simulink model "main"  (R2021a)
settings: Solver=FixedStepDiscrete  StartTime=0  StopTime=20  FixedStep=0.1  RelTol=1e-3
PreLoadFcn:
  | preloadFcn
values from neighbouring files (symbols this model uses):
  egoTargetSpd_kph = 60    [preloadFcn.m]
  iniEgoHeading = egoInfo(1,3)    [preloadFcn.m]
  iniEgoPos = egoInfo(1,1:2)    [preloadFcn.m]
  iniEgoSpd = egoInfo(1,4:5)    [preloadFcn.m]
  iniObsHeading1 = refInfo_obs1(1,3)    [preloadFcn.m]
  iniObsHeading2 = refInfo_obs2(1,3)    [preloadFcn.m]
  iniObsPos1 = refInfo_obs1(1,1:2)    [preloadFcn.m]
  iniObsPos2 = refInfo_obs2(1,1:2)    [preloadFcn.m]
  iniObsSpd1 = refInfo_obs1(1,4:5)    [preloadFcn.m]
  iniObsSpd2 = refInfo_obs2(1,4:5)    [preloadFcn.m]
  mu = [-2.06408447904 -1.49508472185]    [dataSet.mat]
  sig = [50.3880002876 29.2458553231]    [dataSet.mat]
undefined symbols (not defined in the file or in its folder): leftWaypoints, refInfo_obs1, refInfo_obs2, rightWaypoints
libraries: deeplib x2, fuzblock x1
(part 1 of 2)
settings Model: Creator=Ally  LastModifiedBy=Ally

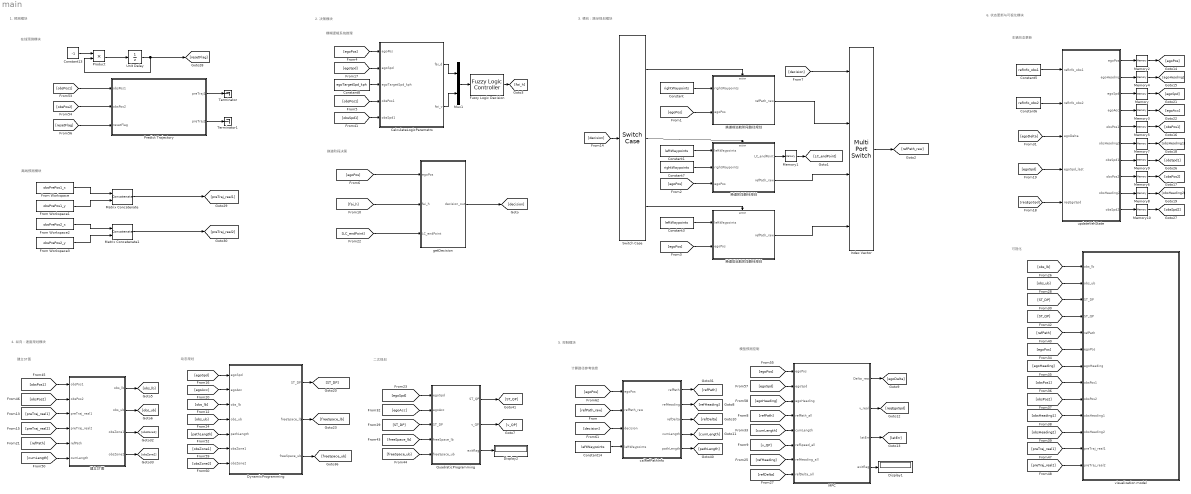
== system main ==
  note: 可视化
  note: 车辆状态更新
  note: 模型预测控制
  note: 计算路径参考信息
  note: 二次规划
  note: 动态规划
  note: 建立ST图
  note: 换道阶段决策
  note: 模糊逻辑系统推理
  note: 在线预测模块
  note: 离线预测模块
  note: 6. 状态更新与可视化模块
  note: 5. 控制模块
  note: 4. 纵向：速度规划模块
  note: 3. 横向：路径规划模块
  note: 2. 决策模块
  note: 1. 预测模块
  CalculateLogicParemetrs : MATLAB Function  TreatAsAtomicUnit=on
  Constant : Constant  Value=rightWaypoints
  Constant1 : Constant  Value=leftWaypoints
  Constant13 : Constant  Value=-1
  Constant14 : Constant  Value=leftWaypoints
  Constant3 : Constant  Value=leftWaypoints
  Constant5 : Constant  Value=refInfo_obs1
  Constant6 : Constant  Value=refInfo_obs2
  Constant7 : Constant  Value=rightWaypoints
  Constant8 : Constant  Value=egoTargetSpd_kph
  Display1 : Display
  Display2 : Display
  DynamicProgramming : MATLAB Function  TreatAsAtomicUnit=on
  From Workspace : FromWorkspace  VariableName=obsPrePos1_x
  From Workspace1 : FromWorkspace  VariableName=obsPrePos1_y
  From Workspace2 : FromWorkspace  VariableName=obsPrePos2_x
  From Workspace3 : FromWorkspace  VariableName=obsPrePos2_y
  Fuzzy Logic Decision : fuzblock/Fuzzy Logic  Controller  FIS='LCD.fis'  OutputSampleNumber=101  DataType=double  FuzzifiedInputs=off  RuleFiringStrengths=off  RuleOutputs=off  AggregatedOutputs=off  SimulateUsing=Interpreted execution  OutOfRangeInputValueMessage=warning  NoRuleFiredMessage=warning  EmptyOutputFuzzySetMessage=warning
  Index Vector : MultiPortSwitch
  MPC : MATLAB Function  TreatAsAtomicUnit=on
  Matrix Concatenate : Concatenate  Mode=Multidimensional array  ConcatenateDimension=2
  Matrix Concatenate1 : Concatenate  Mode=Multidimensional array  ConcatenateDimension=2
  Memory : Memory  InitialCondition=iniEgoSpd
  Memory1 : Memory  InitialCondition=[0 0]
  Memory10 : Memory  InitialCondition=iniObsSpd2
  Memory2 : Memory  InitialCondition=iniEgoPos
  Memory3 : Memory
  Memory4 : Memory  InitialCondition=iniEgoHeading
  Memory5 : Memory  InitialCondition=iniObsPos1
  Memory6 : Memory  InitialCondition=iniObsPos2
  Memory7 : Memory  InitialCondition=iniObsHeading1
  Memory8 : Memory  InitialCondition=iniObsHeading2
  Memory9 : Memory  InitialCondition=iniObsSpd1
  Mux1 : Mux  Inputs=2
  Predict Trajectory : Subsystem  TreatAsAtomicUnit=on
  Product : Product
  QuadraticProgramming : MATLAB Function  TreatAsAtomicUnit=on
  Switch Case : SwitchCase  CaseConditions={1,2,3}  ShowDefaultCase=off
  Terminator : Terminator
  Terminator1 : Terminator
  Unit Delay : UnitDelay  InitialCondition=1  SampleTime=-1  HasFrameUpgradeWarning=on
  calRefPathInfo : MATLAB Function  TreatAsAtomicUnit=on
  getDecision : MATLAB Function  TreatAsAtomicUnit=on
  updateVehState : MATLAB Function  TreatAsAtomicUnit=on
  visualization model : MATLAB Function  TreatAsAtomicUnit=on
  建立ST图 : MATLAB Function  TreatAsAtomicUnit=on
  换道前巡航阶段路径规划 : Subsystem  TreatAsAtomicUnit=on
  换道后巡航阶段路径规划 : Subsystem  TreatAsAtomicUnit=on
  换道阶段路径规划 : Subsystem  TreatAsAtomicUnit=on
  wires:
  CalculateLogicParemetrs/1(fai_d) -> Mux1/1
  [egoPos] -> CalculateLogicParemetrs/1(egoPos)
  getDecision/1(decision_out) -> [decision]
  CalculateLogicParemetrs/2(fai_v) -> Mux1/2
  [egoSpd] -> CalculateLogicParemetrs/2(egoSpd)
  [LC_endPoint] -> getDecision/3(LC_endPoint)
  Mux1/1 -> Fuzzy Logic Decision/1
  Switch Case/2 -> 换道阶段路径规划/Action
  Switch Case/1 -> 换道前巡航阶段路径规划/Action
  [decision] -> Switch Case/1
  Constant/1 -> 换道前巡航阶段路径规划/1(rightWaypoints)
  [egoPos] -> 换道前巡航阶段路径规划/2(egoPos)
  Constant1/1 -> 换道阶段路径规划/1(leftWaypoints)
  [egoPos] -> 换道后巡航阶段路径规划/2(egoPos)
  Constant3/1 -> 换道后巡航阶段路径规划/1(leftWaypoints)
  Switch Case/3 -> 换道后巡航阶段路径规划/Action
  换道前巡航阶段路径规划/1(refPath_raw) -> Index Vector/2
  换道后巡航阶段路径规划/1(refPath_raw) -> Index Vector/4
  [decision] -> Index Vector/1
  Index Vector/1 -> [refPath_raw]
  [preTraj_real1] -> 建立ST图/3(preTraj_real1)
  [preTraj_real2] -> 建立ST图/4(preTraj_real2)
  [refPath] -> 建立ST图/5(refPath)
  建立ST图/1(obs_lb) -> [obs_lb]
  建立ST图/2(obs_ub) -> [obs_ub]
  [obs_lb] -> DynamicProgramming/3(obs_lb)
  [obs_ub] -> DynamicProgramming/4(obs_ub)
  QuadraticProgramming/2(v_QP) -> [v_QP]
  [refPath_raw] -> calRefPathInfo/2(refPath_raw)
  calRefPathInfo/2(refHeading) -> [refHeading]
  calRefPathInfo/3(refDelta) -> [refDelta]
  calRefPathInfo/4(cumLength) -> [cumLength]
  [refPath] -> MPC/4(refPath_all)
  [v_QP] -> MPC/6(refSpeed_all)
  [refHeading] -> MPC/7(refHeading_all)
  [refDelta] -> MPC/8(refDelta_all)
  MPC/1(Delta_real) -> [egoDelta]
  MPC/3(latErr) -> [latErr]
  Constant5/1 -> updateVehState/1(refInfo_obs1)
  Constant6/1 -> updateVehState/2(refInfo_obs2)
  [egoDelta] -> updateVehState/3(egoDelta)
  [reqEgoSpd] -> updateVehState/5(reqEgoSpd)
  updateVehState/1(egoPos) -> Memory2/1
  updateVehState/2(egoHeading) -> Memory4/1
  updateVehState/5(obsPos1) -> Memory5/1
  updateVehState/8(obsPos2) -> Memory6/1
  updateVehState/6(obsHeading1) -> Memory7/1
  updateVehState/9(obsHeading2) -> Memory8/1
  [obs_lb] -> visualization model/1(obs_lb)
  [obs_ub] -> visualization model/2(obs_ub)
  DynamicProgramming/1(ST_DP) -> [ST_DP]
  [ST_DP] -> QuadraticProgramming/3(ST_DP)
  [ST_DP] -> visualization model/3(ST_DP)
  [ST_QP] -> visualization model/4(ST_QP)
  [refPath] -> visualization model/5(refPath)
  [egoPos] -> visualization model/6(egoPos)
  [egoHeading] -> visualization model/7(egoHeading)
  [obsPos1] -> visualization model/8(obsPos1)
  [obsPos2] -> visualization model/9(obsPos2)
  [obsHeading1] -> visualization model/10(obsHeading1)
  [obsHeading2] -> visualization model/11(obsHeading2)
  [egoPos] -> 换道阶段路径规划/3(egoPos)
  [egoPos] -> getDecision/1(egoPos)
  MPC/2(v_real) -> [reqEgoSpd]
  updateVehState/3(egoSpd) -> Memory/1
  updateVehState/4(egoAcc) -> Memory3/1
  Memory/1 -> [egoSpd]
  [egoSpd] -> updateVehState/4(egoSpd_last)
  updateVehState/7(obsSpd1) -> Memory9/1
  updateVehState/10(obsSpd2) -> Memory10/1
  Constant8/1 -> CalculateLogicParemetrs/3(egoTargetSpd_kph)
  [obsPos1] -> CalculateLogicParemetrs/4(obsPos1)
  [obsSpd1] -> CalculateLogicParemetrs/5(obsSpd1)
  Memory1/1 -> [LC_endPoint]
  Memory2/1 -> [egoPos]
  Memory3/1 -> [egoAcc]
  Memory4/1 -> [egoHeading]
  Memory5/1 -> [obsPos1]
  Memory6/1 -> [obsPos2]
  Memory7/1 -> [obsHeading1]
  Memory8/1 -> [obsHeading2]
  Memory9/1 -> [obsSpd1]
  Memory10/1 -> [obsSpd2]
  Constant7/1 -> 换道阶段路径规划/2(rightWaypoints)
  [egoSpd] -> DynamicProgramming/1(egoSpd)
  [egoAcc] -> DynamicProgramming/2(egoAcc)
  [egoAcc] -> QuadraticProgramming/2(egoAcc)
  DynamicProgramming/2(freeSpace_lb) -> [freeSpace_lb]
  DynamicProgramming/3(freeSpace_ub) -> [freeSpace_ub]
  [freeSpace_lb] -> QuadraticProgramming/4(freeSpace_lb)
  [freeSpace_ub] -> QuadraticProgramming/5(freeSpace_ub)
  [egoSpd] -> QuadraticProgramming/1(egoSpd)
  QuadraticProgramming/3(exitflag) -> Display2/1
  calRefPathInfo/5(pathLength) -> [pathLength]
  [cumLength] -> 建立ST图/6(cumLength)
  [pathLength] -> DynamicProgramming/5(pathLength)
  MPC/4(exitflag) -> Display1/1
  QuadraticProgramming/1(ST_QP) -> [ST_QP]
  [cumLength] -> MPC/5(cumLength)
  [obsPos1] -> 建立ST图/1(obsPos1)
  [obsPos2] -> 建立ST图/2(obsPos2)
  [preTraj_real1] -> visualization model/12(preTraj_real1)
  [preTraj_real2] -> visualization model/13(preTraj_real2)
  Product/1 -> Unit Delay/1
  Unit Delay/1 -> [resetFlag], Product/2
  Constant13/1 -> Product/1
  [resetFlag] -> Predict Trajectory/3(resetFlag)
  [obsPos1] -> Predict Trajectory/1(obsPos1)
  [obsPos2] -> Predict Trajectory/2(obsPos2)
  Predict Trajectory/1(preTraj1) -> Terminator/1
  Predict Trajectory/2(preTraj2) -> Terminator1/1
  From Workspace/1 -> Matrix Concatenate/1
  From Workspace1/1 -> Matrix Concatenate/2
  From Workspace2/1 -> Matrix Concatenate1/1
  From Workspace3/1 -> Matrix Concatenate1/2
  Matrix Concatenate/1 -> [preTraj_real1]
  Matrix Concatenate1/1 -> [preTraj_real2]
  [egoPos] -> MPC/1(egoPos)
  [egoSpd] -> MPC/2(egoSpd)
  [egoHeading] -> MPC/3(egoHeading)
  calRefPathInfo/1(refPath) -> [refPath]
  建立ST图/3(obsZone1) -> [obsZone1]
  建立ST图/4(obsZone2) -> [obsZone2]
  [obsZone1] -> DynamicProgramming/6(obsZone1)
  [obsZone2] -> DynamicProgramming/7(obsZone2)
  [decision] -> calRefPathInfo/3(decision)
  [egoPos] -> calRefPathInfo/1(egoPos)
  Constant14/1 -> calRefPathInfo/4(leftWaypoints)
  Fuzzy Logic Decision/1 -> [fai_h]
  [fai_h] -> getDecision/2(fai_h)
  换道阶段路径规划/1(LC_endPoint) -> Memory1/1
  换道阶段路径规划/2(refPath_raw) -> Index Vector/3

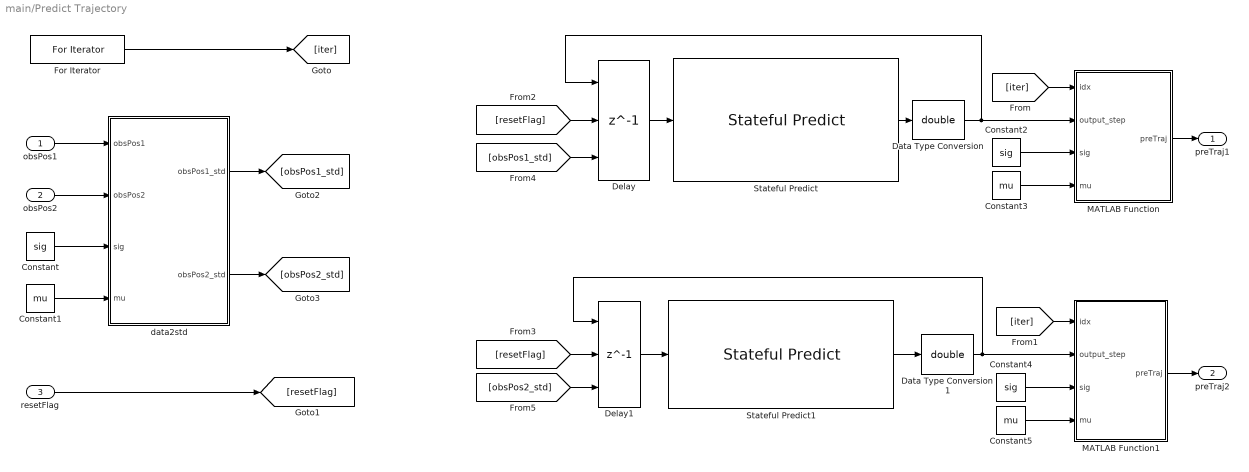
== system main/Predict Trajectory ==
  obsPos1 : Inport
  obsPos2 : Inport  Port=2
  resetFlag : Inport  Port=3
  Constant : Constant  Value=sig
  Constant1 : Constant  Value=mu
  Constant2 : Constant  Value=sig
  Constant3 : Constant  Value=mu
  Constant4 : Constant  Value=sig
  Constant5 : Constant  Value=mu
  Data Type Conversion : DataTypeConversion  OutDataTypeStr=double
  Data Type Conversion1 : DataTypeConversion  OutDataTypeStr=double
  Delay : Delay  DelayLength=1  InitialConditionSource=Input port  ExternalReset=Either
      settings: InputPortMap=u0,r5,p4
  Delay1 : Delay  DelayLength=1  InitialConditionSource=Input port  ExternalReset=Either
      settings: InputPortMap=u0,r5,p4
  For Iterator : ForIterator  IterationLimit=10
  MATLAB Function : MATLAB Function  TreatAsAtomicUnit=on
  MATLAB Function1 : MATLAB Function  TreatAsAtomicUnit=on
  Stateful Predict : deeplib/Stateful Predict  Network=Network from MAT-file  NetworkFunction=untitled  NetworkFilePath=C:\Users\Ally\Desktop\LSTM.mat  InputDataFormats={ '', '' }  SampleTime=-1  ForceInterpretedSim=off  EnableDLNetwork=on
      settings: SourceProductBaseCode=NN
  Stateful Predict1 : deeplib/Stateful Predict  Network=Network from MAT-file  NetworkFunction=untitled  NetworkFilePath=C:\Users\Ally\Desktop\LSTM.mat  InputDataFormats={ '', '' }  SampleTime=-1  ForceInterpretedSim=off  EnableDLNetwork=on
      settings: SourceProductBaseCode=NN
  data2std : MATLAB Function  TreatAsAtomicUnit=on
  preTraj1 : Outport
  preTraj2 : Outport  Port=2
  wires:
  data2std/2(obsPos2_std) -> [obsPos2_std]
  [obsPos2_std] -> Delay1/3
  data2std/1(obsPos1_std) -> [obsPos1_std]
  Constant1/1 -> data2std/4(mu)
  Stateful Predict1/1 -> Data Type Conversion1/1
  obsPos2/1 -> data2std/2(obsPos2)
  For Iterator/1 -> [iter]
  [resetFlag] -> Delay1/2
  Data Type Conversion/1 -> MATLAB Function/2(output_step), Delay/1
  Delay1/1 -> Stateful Predict1/1
  MATLAB Function/1(preTraj) -> preTraj1/1
  Data Type Conversion1/1 -> MATLAB Function1/2(output_step), Delay1/1
  Constant4/1 -> MATLAB Function1/3(sig)
  obsPos1/1 -> data2std/1(obsPos1)
  [iter] -> MATLAB Function/1(idx)
  MATLAB Function1/1(preTraj) -> preTraj2/1
  [iter] -> MATLAB Function1/1(idx)
  resetFlag/1 -> [resetFlag]
  [resetFlag] -> Delay/2
  Constant2/1 -> MATLAB Function/3(sig)
  Constant3/1 -> MATLAB Function/4(mu)
  Constant/1 -> data2std/3(sig)
  Constant5/1 -> MATLAB Function1/4(mu)
  Stateful Predict/1 -> Data Type Conversion/1
  [obsPos1_std] -> Delay/3
  Delay/1 -> Stateful Predict/1

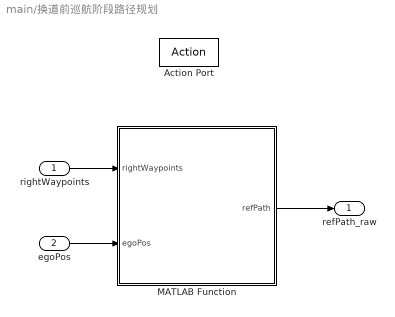
== system main/换道前巡航阶段路径规划 ==
  rightWaypoints : Inport
  egoPos : Inport  Port=2
  Action Port : ActionPort  ActionPortLabel=case [ 1 ]:
  MATLAB Function : MATLAB Function  TreatAsAtomicUnit=on
  refPath_raw : Outport  VectorParamsAs1DForOutWhenUnconnected=off
  wires:
  rightWaypoints/1 -> MATLAB Function/1(rightWaypoints)
  MATLAB Function/1(refPath) -> refPath_raw/1
  egoPos/1 -> MATLAB Function/2(egoPos)

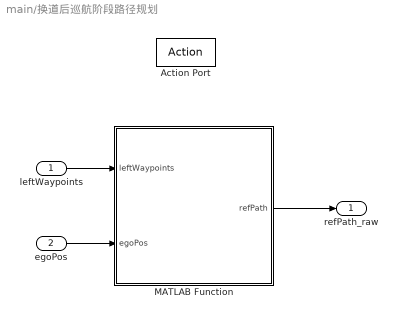
== system main/换道后巡航阶段路径规划 ==
  leftWaypoints : Inport
  egoPos : Inport  Port=2
  Action Port : ActionPort  ActionPortLabel=case [ 3 ]:
  MATLAB Function : MATLAB Function  TreatAsAtomicUnit=on
  refPath_raw : Outport  VectorParamsAs1DForOutWhenUnconnected=off
  wires:
  egoPos/1 -> MATLAB Function/2(egoPos)
  MATLAB Function/1(refPath) -> refPath_raw/1
  leftWaypoints/1 -> MATLAB Function/1(leftWaypoints)

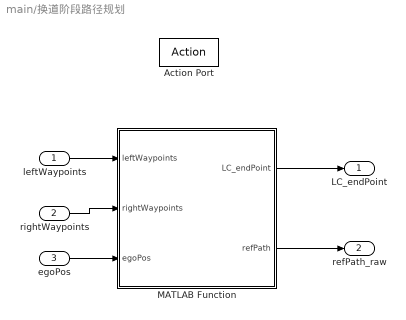
== system main/换道阶段路径规划 ==
  leftWaypoints : Inport
  rightWaypoints : Inport  Port=2
  egoPos : Inport  Port=3
  Action Port : ActionPort  ActionPortLabel=case [ 2 ]:
  MATLAB Function : MATLAB Function  TreatAsAtomicUnit=on
  LC_endPoint : Outport  VectorParamsAs1DForOutWhenUnconnected=off
  refPath_raw : Outport  Port=2  VectorParamsAs1DForOutWhenUnconnected=off
  wires:
  rightWaypoints/1 -> MATLAB Function/2(rightWaypoints)
  leftWaypoints/1 -> MATLAB Function/1(leftWaypoints)
  egoPos/1 -> MATLAB Function/3(egoPos)
  MATLAB Function/1(LC_endPoint) -> LC_endPoint/1
  MATLAB Function/2(refPath) -> refPath_raw/1

== matlab function main/CalculateLogicParemetrs ==
  data: egoPos input; fai_d output; egoSpd input; egoTargetSpd_kph input; obsPos1 input; obsSpd1 input; fai_v output
function [fai_d,fai_v] = CalculateLogicParemetrs(egoPos,egoSpd,egoTargetSpd_kph, obsPos1, obsSpd1)
deltDist = sqrt((egoPos(1)-obsPos1(1))^2 + (egoPos(2)-obsPos1(2))^2);
egoSpd_abs = sqrt(egoSpd(1)^2 + egoSpd(2)^2);
obsSpd_abs = sqrt(obsSpd1(1)^2 + obsSpd1(2)^2);

% 计算安全距离模型
D_slf = (egoSpd_abs-obsSpd_abs)^2 / 2/(0.0524*egoSpd_abs-0.1215) + 0.8509*obsSpd_abs+1.6109;

% 计算车距期望系数
D_f = D_slf + 10;    % 车距期望值
if deltDist >= D_f
    fai_d = 1;
else
    fai_d = deltDist / D_f;
end

% 计算速度差值系数
egoTargetSpd_mps = egoTargetSpd_kph / 3.6;   
if egoSpd_abs >= egoTargetSpd_mps
    fai_v = 1;
else
    fai_v = (egoSpd_abs - obsSpd_abs) / egoTargetSpd_mps;
end

== matlab function main/getDecision ==
  data: egoPos input; fai_h input; decision_out output; LC_endPoint input
function decision_out = getDecision(egoPos,fai_h,LC_endPoint)
persistent flag decision
if isempty(flag) || isempty(decision) 
    flag = 0;
    decision = 1;
end

if fai_h <= 0.5 && decision <= 1
    decision = 1;
else 
    % 计算本车位置与换道终点的距离
    dist = sqrt((egoPos(1) - LC_endPoint(1))^2 + (egoPos(2) - LC_endPoint(2))^2);
    if dist < 1 && flag == 0 || flag == 1
        decision = 3;
        flag = 1;
    else
        decision = 2;
    end
end
decision_out = decision;

== matlab function main/DynamicProgramming ==
  data: egoSpd input; egoAcc input; obs_lb input; ST_DP output; obs_ub input; freeSpace_lb output; freeSpace_ub output; pathLength input; obsZone1 input; obsZone2 input
function [ST_DP,freeSpace_lb,freeSpace_ub] = DynamicProgramming(egoSpd,egoAcc,obs_lb,obs_ub, pathLength, obsZone1, obsZone2)
%% 初始化
% 初始速度和加速度
v_ini = sqrt(egoSpd(1)^2 + egoSpd(2)^2);
a_ini = egoAcc;

% 路径长度限制在100米内
pathLength_max = 100;
pathLength = min([pathLength,pathLength_max]);

% 约束条件
v_max = 16;                % 最大速度
a_max = 3;                 % 最大加速度
omega = [0.4, 0.6];        % 加速度和加加速度权重

% 初始条件判断：若初始速度和加速度不满足上限值，则适当进行强制处理，避免后期QP规划失败
if v_ini + a_ini*1 > v_max
    v_ini = v_max;
    a_ini = 0;
end

% 定义状态空间，用于DP搜索
T = 8;                     % ST图总时间
dt = 1;                    % 时间离散步长
dS = 0.2;                  % 距离离散步长
N = round(T / dt);         % 一共N个阶段

% 构造表征s、t的状态空间
t_seq = 0:dt:T;                     % 时间离散向量
s_seq_max = 0:dS:pathLength_max;    % 最大的距离离散向量
s_seq = 0:dS:pathLength;            % 距离离散向量
rows = length(s_seq_max);           % 状态空间行数
cols = length(t_seq);               % 状态空间列数
validRows = length(s_seq);          % 有效的状态空间行数
stateSpace_t = zeros(rows,cols);
stateSpace_s = zeros(rows,cols);
for i = 1:length(s_seq_max)
    for j = 1:length(t_seq)
        row = length(s_seq_max)-i+1;
        col = j;
        stateSpace_t(row,col) = t_seq(j);
        stateSpace_s(row,col) = s_seq_max(i);
    end
end

%% 第1阶段（时刻0）的初步计算
% 遍历第2阶段，初步生成从第一阶段的起点到第二阶段的所有可能状态
state = zeros(12000,6);
stateNum = 0;
for i = rows:-1:(rows-validRows+1)
    % 计算位置、速度、加速度、加加速度
    s = stateSpace_s(i,2);
    v = s / dt;
    a = (v - v_ini) / dt;
    jerk = (a - a_ini) / dt;
    
    % 若满足速度、加速度约束，则将此状态追加到state中
    if v <= v_max && abs(a) <= a_max
        % 计算加速度和加加速度代价
        accCost = abs(a);
        jerkCost = abs(jerk);
        cost =  accCost*omega(1) + 2*jerkCost*omega(2);
        
        % 将第1阶段行索引、第2阶段行索引、位置、速度、加速度、加加速度、代价值存放在state中
        stateNum = stateNum + 1;
        state(stateNum,1:6) = [rows,i,s,v,a,cost];
    end
end

% 初始化最优序列
optSeq = cell(1000,1);     % 每一阶段至第1阶段的累计最优序列
for i = 1:1000
    optSeq{i,1} = zeros(9,6);
end
for i = 1:stateNum
    optSeq{i,1}(1,:) = state(i,:);
end

%% 从第2阶段（时刻dt）逐步遍历寻优
lastState = state;          % 将上面第1阶段获得的备选可行状态赋值给lastState

% 第1层循环：第i个阶段
for i = 2:N+1
    % 时间和下一可行状态初始化
    t = i-1;
    nextStateTemp = zeros(12000,6);
    stateNum_i = 1;
    lastStateNum = sum(lastState(:,1)~=0);
    
    % 第2层循环：当前第i阶段的第j个可能状态
    for j = 1:lastStateNum
        state_j = zeros(1000,6);
        stateNum_j = 0;
        lastStepIdx = lastState(j,2);
        
        %  第3层循环：第i+1阶段的第k个可能状态
        for k = lastStepIdx:-1:(rows-validRows+1)
            % 计算位置、速度、加速度、加加速度
            s = stateSpace_s(k,(i-1));
            v = (s - lastState(j,3)) / dt;
            a = (v -  lastState(j,4)) / dt;
            jerk = (a -  lastState(j,5)) / dt;
            
            % 若满足速度、加速度、障碍物约束，则将此状态追加到state_j中
            pt1 = [t+1,s];
            pt2 = [t, lastState(j,3)];
            flag = isIN(pt1, pt2, obsZone1,obsZone2);

            if flag == 0 &&  v <= v_max && abs(a) <= a_max
                % 计算代价函数
                accCost = abs(a);
                jerkCost = abs(jerk);
                cost =  accCost*omega(1) + 2*jerkCost*omega(2);
                
                % 将第i阶段行索引、第i+1阶段行索引、位置、速度、加速度、加加速度、代价值存放在state中
                stateNum_j = stateNum_j + 1;
                state_j(stateNum_j,1:6) = [lastStepIdx,k,s,v,a,cost];
            end
        end
        nextStateTemp(stateNum_i:stateNum_i+stateNum_j-1,:) = state_j(1:stateNum_j,:);
        stateNum_i = stateNum_i + stateNum_j;
    end
    
    % 故障判断：若nextStateTemp为空，表明下阶段已无任何可行状态，则执行下一个循环
    if sum(nextStateTemp(:,1)) ~= 0
        % 先将下一阶段的可行状态排序，然后只取非重复行索引序号放进s_Temp
        [~,sortIdx] = sort(nextStateTemp(:,2));
        nextStateTemp = nextStateTemp(sortIdx,:);
        s_Temp = zeros(500,1);
        uniqueNum = length(unique(nextStateTemp(:,2)));
        s_Temp(1:uniqueNum) = unique(nextStateTemp(:,2));
        
        % 由于从第i阶段的若干状态到第i+1阶段的某个状态可能有多个选择，那么应该择优处理
        nextState = zeros(12000,6);
        stateNum = 0;
        for j = 1:uniqueNum
            s = s_Temp(j);                                % 第i+1阶段的s值
            idx = find(nextStateTemp(:,2) == s);          % 找出到底有多少个重复的s值
            [~,minIdx] = min(nextStateTemp(idx,6));       % 若有多个，选择从i阶段到i+1阶段的s值的代价最小的那一个
            stateNum = stateNum + 1;
            nextState(stateNum,:) = nextStateTemp(idx(minIdx),:);
        end
        
        % 将本阶段的所有最优状态序列添加至opt_seq中
        opt_seq_temp = cell(1000,1);     % 每一阶段至第1阶段的累计最优序列
        for j = 1:1000
            opt_seq_temp{j,1} = zeros(9,6);
        end
        for j = 1:stateNum
            lastStepIdx = nextState(j,1);   %来自于上一个阶段的哪一个状态
            for k = 1:size(optSeq,1)
                row_optSeq_k = sum(optSeq{k,1}(:,1)~=0);
                if row_optSeq_k ~= 0 && optSeq{k,1}(row_optSeq_k,2) == lastStepIdx
                    opt_seq_temp{j,1}(1:row_optSeq_k+1,:) = [optSeq{k,1}(1:row_optSeq_k,:);
                        nextState(j,:)];
                    break
                end
            end
        end
        for j = 1:1000
            if j <= stateNum
                optSeq{j,1} = opt_seq_temp{j,1};
            else
                optSeq{j,1} =  zeros(9,6);
            end
        end
        lastState = nextState;
    end
end

%% 找出最优ST曲线
t_opt = (0:1:8)';
s_opt = [0;optSeq{2,1}(1:8,3)];
for i = 2:N+1
    if s_opt(i) == 0
        s_opt(i) = s_opt(i-1);
    end
end
ST_DP = [t_opt, s_opt];

%% 根据DP得到的ST_opt，更新上下界
freeSpace_lb = zeros(N*10,1);
freeSpace_ub = zeros(N*10,1);
for i = 1:size(ST_DP,1)-1
    s_now = ST_DP(i);
    s_next = ST_DP(i+1);
    for j = 1:10
        s = (s_next - s_now)*j/10 + s_now;
        bound = [obs_lb((i-1)*10+j,2:3), obs_ub((i-1)*10+j,2:3), s];
        temp = sort(bound);
        idx = find(temp == s);
        if idx == 1
            freeSpace_lb((i-1)*10+j) = -1000;
            freeSpace_ub((i-1)*10+j) = temp(2);
        elseif  idx == 5
            freeSpace_lb((i-1)*10+j) = temp(4);
            freeSpace_ub((i-1)*10+j) = 1000;
        else
            freeSpace_lb((i-1)*10+j) = temp(idx-1);
            freeSpace_ub((i-1)*10+j) = temp(idx+1);
        end
    end
end
idx1 = freeSpace_lb == inf;
idx2 = freeSpace_lb == -inf;
freeSpace_lb(idx1) = 1000;
freeSpace_lb(idx2) = -1000;
idx1 = freeSpace_ub == inf;
idx2 = freeSpace_ub == -inf;
freeSpace_ub(idx1) = 1000;
freeSpace_ub(idx2) = -1000;


end

%% 函数
function flag = isIN(pt1, pt2, obsZone1,obsZone2)
x = linspace(pt1(1),pt2(1),10);
y = linspace(pt1(2),pt2(2),10);

num1 = sum(obsZone1(:,1) ~= 0);
num2 = sum(obsZone2(:,1) ~= 0);
if num1 >= 4
    temp1 = double(inpolygon(x, y, obsZone1(1:num1,1), obsZone1(1:num1,2)));
else
    temp1 = zeros(1,10);
end
if num2 >= 4
    temp2 = double(inpolygon(x, y, obsZone2(1:num2,1), obsZone2(1:num2,2)));
else
    temp2 = zeros(1,10);
end
if sum(temp1) == 0 && sum(temp2) == 0
    flag = 0;
else
    flag = 1;
end
end

== matlab function main/MPC ==
  data: egoPos input; egoSpd input; egoHeading input; refPath_all input; cumLength input; refSpeed_all input size=[81,2]; Delta_real output; v_real output; refHeading_all input; refDelta_all input; latErr output; exitflag output
function [Delta_real,v_real,latErr,exitflag] = MPC(egoPos, egoSpd, egoHeading, refPath_all,cumLength, refSpeed_all, refHeading_all,refDelta_all)
%% 预处理
% 将需要跟踪的参考路径缩减为realPathNum个点即可（因为滚动跟踪，无需全部加入）
realPathNum = 10;
refPath = refPath_all(1:realPathNum,:);
refHeading = refHeading_all(1:realPathNum);
refDelta = refDelta_all(1:realPathNum);

% 对QP输出的参考速度序列进行插值获得realPathNum个点
temp = refSpeed_all(:,2) * 0.1;
cumlength_QP = cumsum(temp);
refSpeed =  zeros(1,realPathNum);
refSpeed(1) = refSpeed_all(1,2);
for i = 2:realPathNum
    s = cumLength(i);
    for j = 1:80
        if cumlength_QP(j) < s &&  cumlength_QP(j+1) > s
            refSpeed(i) = refSpeed_all(j,2);
        end
    end
end

%% 主程序
dt = 0.1;   % 时间步长
L = 2.9;    % 轴距

% 车辆初始状态定义
refPos = refPath;
iniPos = egoPos;
iniSpd = egoSpd;
iniHeading = egoHeading*pi/180;

% 赋初值
currentPos = iniPos;
currentHeading = iniHeading;

% 控制量
persistent U
if isempty(U)
    U = [0.01;0.01];
end

% 寻找预瞄距离范围内最近路径点
dist = sqrt((refPos(:,1)-currentPos(1)).^2 + (refPos(:,2)-currentPos(2)).^2);
[~,targetIdx] = min(dist);

% 调用MPC控制器
[Delta_real,v_real,latErr,U,exitflag] = MPC_controller(targetIdx,currentPos,currentHeading,refPos,refHeading,refDelta,dt,L,U,refSpeed);

end

function [Delta_real,v_real,latError,U,exitflag] = MPC_controller...
    (targetIdx,currentPos,currentHeading,refPos,refHeading,refDelta,dt,L,U,refSpeed) 

%% MPC预设参数
Nx = 3;         % 状态量的个数
Nu = 2;         % 控制量的个数
Np = 10;        % 预测步长
Nc = 10;        % 控制步长
rau = 10;       % 松弛因子
Q = 100*eye(Np*Nx);      % (Np*Nx) × (Np*Nx)
R = 1*eye(Nc*Nu);        % (Nc*Nu) × (Nc*Nu)

% 控制量约束条件
umin = [-0.2; -0.54];
umax = [0.2; 0.332];
delta_umin = [-0.05; -0.64];
delta_umax = [0.05; 0.64];

%% 原运动学误差状态空间方程的相关矩阵
% 计算参考控制量
v_r = refSpeed(targetIdx);
Delta_r = refDelta(targetIdx);
heading_r = refHeading(targetIdx);

% 实际状态量与参考状态量
X_real = [currentPos(1),currentPos(2),currentHeading];
Xr = [refPos(targetIdx,1), refPos(targetIdx,2), refHeading(targetIdx)];

% 求位置、航向角的误差
x_error  = currentPos(1) - refPos(targetIdx,1);
y_error = currentPos(2) - refPos(targetIdx,2);

% 根据百度Apolo，计算横向误差
latError = y_error*cos(heading_r) - x_error*sin(heading_r);

% a,b两个矩阵
a = [1    0   -v_r*sin(heading_r)*dt;
    0    1   v_r*cos(heading_r)*dt;
    0    0   1];
b = [cos(heading_r)*dt     0;
    sin(heading_r)*dt     0;
    tan(heading_r)*dt/L   v_r*dt/(L * (cos(Delta_r)^2))];

%% 新的状态空间方程的相关矩阵
coder.extrinsic('cell2mat');
% 新的状态量
kesi = zeros(Nx+Nu,1);              % (Nx+Nu) × 1
kesi(1:Nx) = X_real - Xr;
kesi(Nx+1:end) = U;

% 新的A矩阵
A_cell = cell(2,2);
A_cell{1,1} = a;
A_cell{1,2} = b;
A_cell{2,1} = zeros(Nu,Nx);
A_cell{2,2} = eye(Nu);
A = cell2mat(A_cell);           % (Nx+Nu) × (Nx+Nu)

% 新的B矩阵
B_cell = cell(2,1);
B_cell{1,1} = b;
B_cell{2,1} = eye(Nu);
B = cell2mat(B_cell);           % (Nx+Nu) × Nu

% 新的C矩阵
C = [eye(Nx), zeros(Nx, Nu)];   % Nx × (Nx+Nu)

% PHI矩阵
PHI_cell = cell(Np,1);
for i = 1:Np
    PHI_cell{i,1} = zeros(Nx,Nx+Nu);
    PHI_cell{i,1}=C*A^i;  % Nx × (Nx+Nu)
end
PHI = cell2mat(PHI_cell);   % (Nx * Np) × (Nx + Nu)


% THETA矩阵
THETA_cell = cell(Np,Nc);
for i = 1:Np
    for j = 1:Nc
        THETA_cell{i,j} = zeros(Nx,Nu);
        if j <= i
            THETA_cell{i,j} = C*A^(i-j)*B;    % Nx × Nu
        end
    end
end
THETA = zeros(Nx * Np,Nu * Nc);
THETA = cell2mat(THETA_cell);                 % (Nx * Np) × (Nu * Nc)

%% 二次型目标函数的相关矩阵

% 初始化H矩阵
H_cell = cell(2,2);
H_cell{1,1} = zeros(Nu*Nc, Nu*Nc);
H_cell{1,1} = THETA'*Q*THETA + R;  % (Nu * Nc) × (Nu * Nc)
H_cell{1,2} = zeros(Nu*Nc,1);
H_cell{2,1} = zeros(1,Nu*Nc);
H_cell{2,2} = rau;
H = cell2mat(H_cell);            % (Nu * Nc + 1) × (Nu * Nc + 1)

% E矩阵
E = PHI*kesi;                    % (Nx * Np) × 1

% g矩阵
g_cell = cell(2,1);
g_cell{1,1} = zeros(Nu * Nc,1);
g_cell{1,1} = E'*Q*THETA;          % (Nu * Nc ) × 1，行数为了和H的列数匹配，新添加一列0
g_cell{2,1} = 0;
g = cell2mat(g_cell);              % (Nu * Nc + 1 ) × 1

%% 约束条件的相关矩阵

% A_I矩阵
A_t = zeros(Nc,Nc);     % 下三角方阵
for i = 1:Nc
    A_t(i,1:i) = 1;
end
A_I = kron(A_t,eye(Nu));       % (Nu * Nc) × (Nu * Nc)

% Ut矩阵
Ut = kron(ones(Nc,1),U);       % (Nu * Nc) × 1

% 控制量与控制量变化量的约束
Umin = kron(ones(Nc,1),umin);
Umax = kron(ones(Nc,1),umax);
delta_Umin = kron(ones(Nc,1),delta_umin);
delta_Umax = kron(ones(Nc,1),delta_umax);

% 用于quadprog函数不等式约束Ax <= b的矩阵A
A_cons_cell = {A_I, zeros(Nu*Nc,1);       % 列数为了和H的列数匹配，新添加一列0，(Nu * Nc) × (Nu * Nc), (Nu * Nc) ×1
    -A_I, zeros(Nu*Nc,1)};
A_cons = cell2mat(A_cons_cell);           % (Nu * Nc * 2) × (Nu * Nc +1)

% 用于quadprog函数不等式约束Ax <= b的向量b
b_cons_cell = {Umax-Ut;
    -Umin+Ut};
b_cons = cell2mat(b_cons_cell);

% △U的上下界约束
lb = [delta_Umin;0];
ub = [delta_Umax;0];

%% 开始求解过程
options = optimoptions('quadprog','algorithm','active-set');
exitflag = 0;
delta_U = zeros((Nu * Nc +1),1);
x0 = zeros(Nu * Nc +1,1);
[delta_U,~,exitflag,~]  = quadprog(H,g,A_cons,b_cons,[],[],lb,ub,x0,options);   %(Nu * Nc +1) × 1

%% 计算输出

% 只选取求解的delta_U的第一组控制量。注意：这里是v_tilde的变化量和Delta_tilde的变化量
delta_v_tilde = delta_U(1);
delta_Delta_tilde = delta_U(2);

% 更新这一时刻的控制量。注意，这里的“控制量”是v_tilde和Delta_tilde，而不是真正的v和Delta
U(1) = kesi(4) + delta_v_tilde;
U(2) = kesi(5) + delta_Delta_tilde;

% 求解真正的控制量v_real和Delta_real
v_real = U(1) + v_r;
Delta_real = U(2) + Delta_r;
kk=1;
end

== matlab function main/calRefPathInfo ==
  data: egoPos input; refPath output; refPath_raw input; refHeading output; refDelta output; cumLength output; pathLength output size=1; decision input; leftWaypoints input
function [refPath,refHeading,refDelta,cumLength,pathLength] = calRefPathInfo(egoPos, refPath_raw, decision, leftWaypoints)
%% 相关参数定义
L = 2.9;    % 轴距

% 定义参考轨迹：若决策为2，表明处于换道阶段，需要对轨迹进行简单处理
if decision == 2
    % 第一部分
    deltX = refPath_raw(:,1) - egoPos(1);
    deltY = refPath_raw(:,2) - egoPos(2);
    dist = sqrt(deltX.^2 + deltY.^2);
    [~, idx1] = min(dist);
    refPath = zeros(40,2);
    refPath(1:40-idx1+1,:) = refPath_raw(idx1:40,:);
    
    % 第二部分
    if idx1 >= 2
        LC_endPoint = refPath_raw(40,:);
        deltX = leftWaypoints(:,1) - LC_endPoint(1);
        deltY = leftWaypoints(:,2) - LC_endPoint(2);
        dist = sqrt(deltX.^2 + deltY.^2);
        [~, idx2] = min(dist);
        refPath(40-idx1+2:40,:) = leftWaypoints(idx2+1 :idx1+idx2-1,1:2);
    end
else
    refPath = refPath_raw;
end
    
% 计算航向角
realPathNum = 40;
diff_x = diff(refPath(1:realPathNum,1)) ;
diff_y = diff(refPath(1:realPathNum,2)) ;
cumLength = [0;cumsum(sqrt(diff_x.^2 + diff_y.^2))];
pathLength = sum(sqrt(diff_x.^2 + diff_y.^2));
refHeading = zeros(1,200);
refHeading(1:realPathNum-1) = atan2(diff_y(1:realPathNum-1) , diff_x(1:realPathNum-1));                   % 航向角
refHeading(realPathNum) = refHeading(realPathNum-1);

% 曲率
refCur = zeros(1,realPathNum);
for i = 1:realPathNum
    if i <= realPathNum-2
        x = refPath(i:i+2,1);
        y = refPath(i:i+2,2);
        refCur(i) = getCur(x,y);
    else
        refCur(i) = refCur(realPathNum-2);
    end
end

% 根据阿克曼转向原理，计算参考前轮转角
refDelta = atan(L*refCur);
end

%% 函数
function k=getCur(x,y)
ta=sqrt((x(2)-x(1))^2+(y(2)-y(1))^2);
tb=sqrt((x(3)-x(2))^2+(y(3)-y(2))^2);
M=[1,-ta,ta^2;
    1,0,0;
    1,tb,tb^2];
A=M\x;
B=M\y;
k=(2*(A(2)*B(3)-A(3)*B(2)))/((A(2)^2+B(2)^2)^1.5+1e-10);
end

== matlab function main/updateVehState ==
  data: refInfo_obs1 input; refInfo_obs2 input; egoPos output; egoHeading output; egoSpd output; egoAcc output; obsPos1 output; obsHeading1 output; obsSpd1 output; obsPos2 output; egoDelta input; egoSpd_last input; reqEgoSpd input; obsHeading2 output; obsSpd2 output
function [egoPos,egoHeading,egoSpd,egoAcc,obsPos1,obsHeading1,obsSpd1,obsPos2, obsHeading2,obsSpd2]  = ...
    updateVehState(refInfo_obs1, refInfo_obs2,egoDelta, egoSpd_last, reqEgoSpd)
% 参数
L = 2.9;
dt = 0.1;

% 定义静态变量、初始化
persistent  pos_ego pos_obs1 pos_obs2 obsPosIdx1 obsPosIdx2 heading_ego heading_obs1 heading_obs2
if isempty(pos_ego) || isempty(heading_ego) || isempty(pos_obs1) || isempty(pos_obs2)...
        || isempty(obsPosIdx1) || isempty(obsPosIdx2) || isempty(heading_obs1) || isempty(heading_obs2)
    heading_ego = -129*pi/180;
    obsPosIdx1 = 1;
    obsPosIdx2 = 1;
    pos_ego = [-52.3719, 49.9983];
end

% 本车状态更新
egoSpd = zeros(1,2);
egoSpd(1) = reqEgoSpd * cos(heading_ego);
egoSpd(2) = reqEgoSpd * sin(heading_ego);
egoSpd_last_abs = sqrt(egoSpd_last(1)^2 + egoSpd_last(2)^2);
egoAcc = (reqEgoSpd - egoSpd_last_abs) / 0.1;
max_steer = 60 * pi/180;
egoDelta = max(min(max_steer, egoDelta), -max_steer);
heading_ego = heading_ego + reqEgoSpd / L * tan(egoDelta) * dt ;
pos_ego(1) = pos_ego(1) + egoSpd(1) * dt;
pos_ego(2) = pos_ego(2) + egoSpd(2) * dt;
egoHeading = heading_ego*180/pi;
egoPos = pos_ego;


% 1号交通车状态更新
obsPosIdx1 = obsPosIdx1+1;
pos_obs1 = refInfo_obs1(obsPosIdx1,1:2);
heading_obs1 = refInfo_obs1(obsPosIdx1,3);
obsPos1 = pos_obs1;
obsSpd1 = refInfo_obs1(obsPosIdx1,4:5);
obsHeading1 = heading_obs1;


% 2号交通车状态更新
obsPosIdx2 = obsPosIdx2+1;
pos_obs2 = refInfo_obs2(obsPosIdx2,1:2);
heading_obs2 = refInfo_obs2(obsPosIdx2,3);
obsPos2 = pos_obs2;
obsSpd2 = refInfo_obs2(obsPosIdx2,4:5);
obsHeading2 = heading_obs2;
end

== matlab function main/visualization model ==
  data: obs_lb input; obs_ub input; ST_DP input; ST_QP input; refPath input; egoPos input; egoHeading input; obsPos1 input; obsPos2 input; obsHeading1 input; obsHeading2 input; preTraj_real1 input; preTraj_real2 input
function visualization(obs_lb, obs_ub, ST_DP, ST_QP,refPath, egoPos, egoHeading, obsPos1, obsPos2, obsHeading1, obsHeading2, preTraj_real1, preTraj_real2)
%% 免编译声明
coder.extrinsic('fill');
coder.extrinsic('drivingScenario');
coder.extrinsic('laneMarking');
coder.extrinsic('lanespec');
coder.extrinsic('road');
coder.extrinsic('vehicle');
coder.extrinsic('advance');
coder.extrinsic('trajectory');
coder.extrinsic('findobj');
coder.extrinsic('delete');

%% ST图及DP、QP曲线
obsZone1 = zeros(160,2);
obsZone2 = zeros(160,2);

% 下边界
num1 = 0;
num2 = 0;
for i = 1:81
    t = (i-1)*0.1;
    if ~isinf(obs_lb(i,2))
        num1 = num1 + 1;
        obsZone1(num1,:) = [t,obs_lb(i,2)];
    end
    if ~isinf(obs_lb(i,3))
        num2 = num2 + 1;
        obsZone2(num2,:) = [t,obs_lb(i,3)];
    end
end

% 上边界
for i = 81:-1:1
    t = (i-1)*0.1;
    if ~isinf(obs_ub(i,2))
        num1 = num1 + 1;
        obsZone1(num1,:) = [t,obs_ub(i,2)];
    end
    if ~isinf(obs_ub(i,3))
        num2 = num2 + 1;
        obsZone2(num2,:) = [t,obs_ub(i,3)];
    end
end

figure(1)
clf
fill(obsZone1(1:num1,1), obsZone1(1:num1,2), 'b')
hold on
fill(obsZone2(1:num2,1), obsZone2(1:num2,2), 'b')
plot(ST_DP(:,1),ST_DP(:,2),'g-*');
plot(ST_QP(:,1),ST_QP(:,2),'r.');
grid on
xlim([0,8]);
ylim([0,60]);
xlabel('time / s')
ylabel('distance / m')

%% 场景图

persistent scenario ax2
if isempty(scenario)
    scenario = drivingScenario('SampleTime',0.1);   % 初始化场景
    
    % 道路中心坐标
    roadCenters = [-50 50 0; -50 -50 0; 0 0 0; 50 50 0; 50 -50 0];
    
    % 建立道路
    marking = [laneMarking('Solid') ...
        laneMarking('Dashed') laneMarking('Solid')];             % 分界线线型
    laneSpecification = lanespec(2, 'Marking', marking);         % 道路规范
    road(scenario, roadCenters, 'Lanes', laneSpecification);     % 生成道路
    plot(scenario)
    hold on
    ax2 = gca;
end

% 清除线段句柄
h = findobj('type','Patch','tag','flag1');
delete(h)
h = findobj('type','line','tag','flag2');
delete(h)
h = findobj('type','Patch','tag','flag3');
delete(h)
h = findobj('type','line','tag','flag4');
delete(h)
h = findobj('type','Patch','tag','flag5');
delete(h)
h = findobj('type','line','tag','flag6');
delete(h)

% 画本车矩形框及参考路径
egoProfile = getVehProfile(egoHeading,egoPos);
fill(ax2,egoProfile(:,1),egoProfile(:,2),'k','tag','flag1');
idx = refPath(:,1) ~= 0;
refPath_real = refPath(idx,:);
plot(ax2,refPath_real(:,1),refPath_real(:,2),'r','tag','flag2')

% 画1号交通车矩形框及预测路径
obsProfile1 = getVehProfile(obsHeading1,obsPos1);
fill(ax2,obsProfile1(:,1),obsProfile1(:,2),'k','tag','flag3');
plot(ax2,preTraj_real1(:,1),preTraj_real1(:,2),'k','tag','flag4');

% 画2号交通车矩形框及预测路径
obsProfile2 = getVehProfile(obsHeading2,obsPos2);
fill(ax2,obsProfile2(:,1),obsProfile2(:,2),'k','tag','flag5');
plot(ax2,preTraj_real2(:,1),preTraj_real2(:,2),'k','tag','flag6');


%% 函数
function vehProfile = getVehProfile(heading,frontPos)
% 根据车尾中心点位置和航向角计算车头中心点位置
vehLength = 4.7;
vehWidth = 1.8;
vehHalfWidth = vehWidth/2;
heading = heading * pi/180;

frontPosX = frontPos(1);
frontPosY = frontPos(2);
rearPosX = frontPosX- vehLength * cos(heading);
rearPosY = frontPosY- vehLength * sin(heading);

% 根据前后中心点、航向角计算目障碍车四个轮廓点位置（顺时针编号）
% 每一行代表一个车辆一个角的纵向和横向位置
vehProfile = zeros(4,2);
vehProfile(1,1) = rearPosX - vehHalfWidth * sin(heading);
vehProfile(1,2) = rearPosY + vehHalfWidth * cos(heading);
vehProfile(2,1) = frontPosX - vehHalfWidth * sin(heading);
vehProfile(2,2) = frontPosY + vehHalfWidth * cos(heading);
vehProfile(3,1) = frontPosX + vehHalfWidth * sin(heading);
vehProfile(3,2) = frontPosY - vehHalfWidth * cos(heading);
vehProfile(4,1) = rearPosX + vehHalfWidth * sin(heading);
vehProfile(4,2) = rearPosY - vehHalfWidth * cos(heading);
end
end

== matlab function main/Predict Trajectory/MATLAB Function ==
  data: idx input; preTraj output; output_step input; sig input; mu input
function preTraj = fcn(idx, output_step, sig, mu)
persistent output
if isempty(output)
    output = zeros(2,80);
end
for i = 1:2
    output(i,idx) = sig(i)*output_step(i,10) + mu(i);
    output(i,idx) = sig(i)*output_step(i,10) + mu(i);
end
preTraj = output;

== matlab function main/Predict Trajectory/MATLAB Function1 ==
  data: idx input; preTraj output; output_step input; sig input; mu input
function preTraj = fcn(idx, output_step, sig, mu)
persistent output
if isempty(output)
    output = zeros(2,80);
end
for i = 1:2 
   output(i,idx) = sig(i)*output_step(i,10) + mu(i);
    output(i,idx) = sig(i)*output_step(i,10) + mu(i);
end
preTraj = output;

== matlab function main/Predict Trajectory/data2std ==
  data: obsPos1 input; obsPos1_std output; obsPos2 input; obsPos2_std output; sig input; mu input
function [obsPos1_std, obsPos2_std] = data2std(obsPos1, obsPos2, sig, mu)
% 原始数据转为标准值数据
obsPos1_std = zeros(2,10);
obsPos2_std = zeros(2,10);
for i = 1:2
    obsPos1_std(i,:) = (obsPos1(i,:) - mu(i)) ./ sig(i);
    obsPos2_std(i,:) = (obsPos2(i,:) - mu(i)) ./ sig(i);
end

== matlab function main/换道前巡航阶段路径规划/MATLAB Function ==
  data: refPath output; rightWaypoints input; egoPos input size=[1 2]
function refPath = getRefPath(rightWaypoints, egoPos)
% 计算本车当前位置与右车道中心线最薄距离的索引
deltX = rightWaypoints(:,1) - egoPos(1);
deltY = rightWaypoints(:,2) - egoPos(2);
dist = sqrt(deltX.^2 + deltY.^2);
[~, idx] = min(dist);

% 构造40个参考点
refPath = zeros(40,2);
refPath(1:40,1:2) = rightWaypoints(idx+1:idx+40,1:2);
end

== matlab function main/换道阶段路径规划/MATLAB Function ==
  data: LC_endPoint output; leftWaypoints input; refPath output; rightWaypoints input; egoPos input
function [LC_endPoint,refPath] = fcn(leftWaypoints, rightWaypoints, egoPos)
% 定义path_opt静态变量，用于长期保存所规划的换道路径
% 如此，可以实现每一次进本模块仅需调用，不需重新规划一次
persistent path_opt
if isempty(path_opt)    
    % 计算车辆当前位置在右车道中心线的索引
    deltX = rightWaypoints(:,1) - egoPos(1);
    deltY = rightWaypoints(:,2) - egoPos(2);
    dist = sqrt(deltX.^2 + deltY.^2);
    [~, idx] = min(dist);
    
    % 初始化
    idx_A = idx;
    path = cell(5,5);
    for i = 1:5
        for j = 1:5
            path{i,j} = zeros(40,2);
        end
    end
    totalLength = zeros(5,5);
    mranCur = zeros(5,5);
    cur = zeros(1,40);
    
    % 两层for循环
    for idx_O = idx_A+11 : idx_A+15
        for idx_C = idx_A+4 : idx_A+8
            idx_F =  2*idx_O - idx_A;
            idx_D =  idx_F - (idx_C - idx_A);
            
            % 控制点
            P1 = rightWaypoints(idx_A,1:2);
            P3 = rightWaypoints(idx_C,1:2);
            P4 = leftWaypoints(idx_D,1:2);
            P6 = leftWaypoints(idx_F,1:2);
            P2 = (P1 + P3)/2;
            P5 = (P4 + P6)/2;
            P = [P1; P2; P3; P4; P5; P6]';
            
            % 调用函数生成6控制点3次准均匀B样条曲线
            row = idx_O - idx_A - 10;
            col = idx_C - idx_A -3;
            path{row,col} = B_spline_func(P,5,3);
            
            % 计算路径的路径长度评价函数
            X_r = path{row,col}(:,1);
            Y_r = path{row,col}(:,2);
            diffX = diff(X_r);
            diffY = diff(Y_r);
            deltDist = sqrt(diffX.^2 + diffY.^2);
            totalLength(row,col) = sum(deltDist);
            
            % 计算路径的平均曲率
            for i = 1:length(X_r)-2
                cur(i) = getCur(X_r(i:i+2),Y_r(i:i+2));
            end
            cur(39:40) = cur(40);
            mranCur(row,col) = mean(abs(cur));
        end
    end
     
    % 单独取出路径长度、曲率、曲率变化率三个分代价值
    f1 = totalLength;
    f2 = mranCur;
    
    % 根据权重系数，构造综合目标函数
    f1_norm = std(f1(:));
    f2_norm = std(f2(:));
    alpha = [0.3 0.7];
    f_all = alpha(1)*f1_norm + alpha(2)*f2_norm;
    
    % 求解综合代价函数的最小值的索引，从而获得控制点
    [~,idx] = min(f_all(:));
    [row,col] = ind2sub([5, 5],idx);  
    path_opt = path{row,col};
end
refPath = path_opt;
LC_endPoint = path_opt(40,:);   % 换道路径的终点
end

%% 函数
function B_spline_p = B_spline_func(P,n,k)
B_spline_p=zeros(40,2);
Nik = zeros(n+1, 1);
NodeVector = U_quasi_uniform(n, k); % 准均匀B样条的节点矢量
idx = 0;
for u = 0 : 0.025 : 1-0.025
    for i = 0 : 1 : n
        Nik(i+1, 1) = BaseFunction(i, k , u, NodeVector);
    end
    p_u = P * Nik;
    idx = idx + 1;
    B_spline_p (idx,:)=[p_u(1,1),p_u(2,1)];
end
end

function Nik_u = BaseFunction(i, k , u, NodeVector)
% 计算基函数Ni,k(u),NodeVector为节点向量
if k == 0       % 0次B样条
    if (u >= NodeVector(i+1)) && (u < NodeVector(i+2))
        Nik_u = 1.0;
    else
        Nik_u = 0.0;
    end
else
    Length1 = NodeVector(i+k+1) - NodeVector(i+1);
    Length2 = NodeVector(i+k+2) - NodeVector(i+2);      % 支撑区间的长度
    if Length1 == 0.0       % 规定0/0 = 0
        Length1 = 1.0;
    end
    if Length2 == 0.0
        Length2 = 1.0;
    end
    Nik_u = (u - NodeVector(i+1)) / Length1 * BaseFunction(i, k-1, u, NodeVector) ...
        + (NodeVector(i+k+2) - u) / Length2 * BaseFunction(i+1, k-1, u, NodeVector);
end
end


function NodeVector = U_quasi_uniform(n, k)
% 准均匀B样条的节点向量计算，共n+1个控制顶点，k次B样条，k+1阶
NodeVector = zeros(1, n+k+2);
piecewise = n - k + 1;       % 曲线的段数
if piecewise == 1       % 只有一段曲线时，n = k
    for i = k+2 : n+k+2
        NodeVector(1, i) = 1;
    end
else
    flag = 1;       % 不止一段曲线时
    while flag ~= piecewise
        NodeVector(1, k+1+flag) = NodeVector(1, k + flag) + 1/piecewise;
        flag = flag + 1;
    end
    NodeVector(1, n+2 : n+k+2) = 1;
end
end

% 求曲率
function k=getCur(x,y)
ta=sqrt((x(2)-x(1))^2+(y(2)-y(1))^2);
tb=sqrt((x(3)-x(2))^2+(y(3)-y(2))^2);
M=[1,-ta,ta^2;
    1,0,0;
    1,tb,tb^2];
A=M\x;
B=M\y;
k=(2*(A(2)*B(3)-A(3)*B(2)))/((A(2)^2+B(2)^2)^1.5+1e-10);
end

% 转化为0~1的标准值
function y_std = std(x)
ymin = 0;
ymax = 1;
xmin = min(x);
xmax = max(x);
y_std = (ymax-ymin)*(x-xmin)/(xmax-xmin) + ymin;
end

== matlab function main/换道后巡航阶段路径规划/MATLAB Function ==
  data: refPath output; leftWaypoints input; egoPos input size=[1 2]
function refPath = getRefPath(leftWaypoints, egoPos)
% 计算本车当前位置与左车道中心线最薄距离的索引
deltX = leftWaypoints(:,1) - egoPos(1);
deltY = leftWaypoints(:,2) - egoPos(2);
dist = sqrt(deltX.^2 + deltY.^2);
[~, idx] = min(dist);

% 构造40个参考点
refPath = zeros(40,2);
refPath(1:40,1:2) = leftWaypoints(idx+1:idx+40,1:2);
end

== matlab function main/QuadraticProgramming ==
  data: ST_QP output; egoSpd input; egoAcc input; ST_DP input size=[9,2]; freeSpace_lb input; v_QP output; freeSpace_ub input; exitflag output
function [ST_QP,v_QP,exitflag] = QuadraticProgramming(egoSpd,egoAcc,ST_DP, freeSpace_lb,freeSpace_ub)
%% 参数初始化
% 初始速度和加速度
v_ini = sqrt(egoSpd(1)^2 + egoSpd(2)^2);
a_ini = egoAcc;

% 性能函数指标权重
w1 = 1;    % 加速度权重
w2 = 10;     % 加加速度权重
w3 = 1;      % 与动态规划得到的最优ST曲线的误差指标权重

% DP和QP的离散时间和阶段数量
deltT_DP = 1;
deltT_QP = 0.1;
N_DP = 8;
N_QP = deltT_DP / deltT_QP;

% 约束
v_max = 16;         % 最大速度
v_min = 0;          % 最小速度
acc_max = 3;        % 最大加速度
acc_min = -3;       % 最小加速度

% 初始条件判断：若初始速度和加速度不满足上限值，则适当进行强制处理，避免QP规划失败
if v_ini + a_ini*deltT_QP > v_max
    v_ini = v_max;
    a_ini = 0;
end
%% 目标函数
H = zeros(6*N_DP);      % 初始化H矩阵
f = zeros(6*N_DP,1);    % 初始化f矩阵
t = deltT_DP;           % 每一段5次曲线的终点时刻 
for i = 1:N_DP
    % 加速度指标
    H1 = 2 * [0       0         0         0            0             0
        0       0         0         0            0             0
        0       0        4*t       6*t^2        8*t^3        10*t^4
        0       0       6*t^2      12*t^3      18*t^4        24*t^5
        0       0       8*t^3      18*t^4    (144/5)*t^5     40*t^6
        0       0      10*t^4      24*t^5      40*t^6     (400/7)*t^6
        ];
    
    % 加加速度指标
    H2 = 2 * [0       0         0         0            0             0
        0       0         0         0            0             0
        0       0         0         0            0             0
        0       0         0       36*t         72*t^2        120*t^3
        0       0         0      72*t^2       192*t^3        360*t^4
        0       0         0     120*t^3       360*t^4        720*t^5
        ];
    
    % 与动态规划得到的最优ST曲线的误差指标
    H3 = 2 * [1       t       t^2       t^3         t^4           t^5
        t       t^2      t^3       t^4          t^5           t^6
        t^2     t^3      t^4       t^5          t^6           t^7
        t^3     t^4      t^5       t^6          t^7           t^8
        t^4     t^5      t^6       t^7          t^8           t^9
        t^5     t^6      t^7       t^8          t^9           t^10];
    
    % 将上述计算的各性能指标按照权重相加，构造H矩阵
    idx1 = (i-1)*6+1;
    idx2 = i*6;
    tempH = w1 * H1 + w2 * H2 + w3 * H3;
    H(idx1:idx2, idx1:idx2) = H(idx1:idx2, idx1:idx2) + tempH;
    
    % 由于“与期望的S误差”会产生f项，在此添加
    refS = ST_DP(i+1,2);
    tempF = -2 * refS * [1       t       t^2       t^3         t^4           t^5]' *w3;
    f(idx1:idx2) = f(idx1:idx2) + tempF;
    
end

%% 等式约束
% 每一段的邻接连接点约束：位置、速度、加速度、加加速度约束
Aeq1 = zeros(4*(N_DP-1), 6*N_DP);
Beq1 = zeros(4*(N_DP-1),1);
for i = 1:N_DP-1
    t = deltT_DP;
    % 位置
    aeq1 = [1  t   t^2       t^3       t^4       t^5      -1    0    0   0    0   0];
    % 速度
    aeq2 = [0  1   2*t      3*t^2     4*t^3     5*t^4      0   -1    0   0    0   0];
    % 加速度
    aeq3 = [0  0    2        6*t      12*t^2    20*t^3     0    0   -2   0    0   0];
    % 加加速度
    aeq4 = [0  0    0         6        24*t     60*t^2     0    0   0   -6    0   0];
    
    % b向量
    beq = [0 0 0 0]';
    
    % 将此段约束量添加到大矩阵中
    startRow = (i-1)*4+1;
    endRow = i*4;
    startCol = (i-1)*6+1;
    endCol = (i+1)*6;
    Aeq1(startRow:endRow, startCol:endCol) = [aeq1; aeq2; aeq3; aeq4];
    Beq1(startRow:endRow,1) = beq;
end

% ST曲线起点:位置、速度、加速度约束
Aeq2 = zeros(3,6*N_DP);
Beq2 = zeros(3,1);
t = 0;
aeq1 = [1  t   t^2       t^3       t^4       t^5];
aeq2 = [0  1   2*t      3*t^2     4*t^3     5*t^4];
aeq3 = [0  0    2        6*t      12*t^2    20*t^3];
beq = [ST_DP(1,2), v_ini,  a_ini]';
Aeq2(1:3, 1:6) = [aeq1; aeq2; aeq3];
Beq2(1:3) = beq;

% 组建等式约束矩阵
Aeq = [Aeq1; Aeq2];
Beq = [Beq1; Beq2];

%% 线性不等式约束
% ST图的障碍物上下边界约束
A1 = zeros(N_DP*N_QP*2, 6*N_DP);
B1 = zeros(N_DP*N_QP*2, 1);
for i = 1:N_DP
    for j = 1:N_QP
        t = j*0.1;
        
        % 上下边界
        lb = freeSpace_lb((i-1)*N_QP+j);
        ub = freeSpace_ub((i-1)*N_QP+j)-2;
        
        % 构造Ax ≤b
        a1 = [-1      -t       -t^2      -t^3      -t^4      -t^5];
        a2 = [1       t        t^2       t^3       t^4       t^5];
        b = [-lb ub]';
        
        % 行列索引
        startRow = (i-1)*2*N_QP + (j-1)*2+1;
        endRow = (i-1)*2*N_QP + j*2;
        startCol = (i - 1) * 6 + 1;
        endCol = i * 6;
        
        % 添加到A、B大矩阵中
        A1(startRow:endRow, startCol:endCol) = [a1; a2];
        B1(startRow:endRow,1) = b;
    end
end


% 速度约束
A2 = zeros(N_DP*N_QP*2, 6*N_DP);
B2 = zeros(N_DP*N_QP*2, 1);
for i = 1:N_DP
    for j = 1:N_QP
        t = j*0.1;
        
        % 上下边界
        lb = v_min;
        ub = v_max;
        
        % 构造Ax ≤b
        a1 = [ 0       -1        -2*t      -3*t^2     -4*t^3     -5*t^4];
        a2 = [0       1        2*t      3*t^2     4*t^3     5*t^4];
        b = [-lb ub]';
        
        % 行列索引
        startRow = (i-1)*2*N_QP + (j-1)*2+1;
        endRow = (i-1)*2*N_QP + j*2;
        startCol = (i - 1) * 6 + 1;
        endCol = i * 6;
        
        % 添加到A、B大矩阵中
        A2(startRow:endRow, startCol:endCol) = [a1; a2];
        B2(startRow:endRow,1) = b;
    end
end

% 加速度约束
A3 = zeros(N_DP*N_QP*2, 6*N_DP);
B3 = zeros(N_DP*N_QP*2, 1);
for i = 1:N_DP
    for j = 1:N_QP
        t = j*0.1;
        
        % 上下边界
        lb = acc_min;
        ub = acc_max;
        
        % 构造Ax ≤b
        a1 = [ 0       0       -2        -6*t       -12*t^2     -20*t^3];
        a2 = [0       0        2         6*t        12*t^2      20*t^3];
        b = [-lb ub]';
        
        % 行列索引
        startRow = (i-1)*2*N_QP + (j-1)*2+1;
        endRow = (i-1)*2*N_QP + j*2;
        startCol = (i - 1) * 6 + 1;
        endCol = i * 6;
        
        % 添加到A、B大矩阵中
        A3(startRow:endRow, startCol:endCol) = [a1; a2];
        B3(startRow:endRow,1) = b;
    end
end

% 组建不等式约束矩阵
A = [A1; A2; A3];
B = [B1; B2; B3];

%  调用QP算法
x0 = zeros(1,48);
options = optimoptions('quadprog','algorithm','active-set');
[x,~,exitflag,~] = quadprog(H,f,A,B,Aeq,Beq,[],[],x0,options);

%% 将得到的解x重新调整为N_DP段
ST_QP = zeros(N_DP*N_QP+1, 2);
v_QP = zeros(N_DP*N_QP+1, 2);
a_QP = zeros(N_DP*N_QP+1, 2);

coeff = reshape(x,6,N_DP)';
for i = 1:N_DP
    if i == 1
        ST_QP(1,1) = 0;
        ST_QP(1,2) = ST_DP(1,2);
        v_QP(1,1) = 0;
        v_QP(1,2) = v_ini;
    end
    for j = 1:N_QP
        idx = (i-1)*N_QP + j+1;
        t = j*deltT_QP;
        T = (i-1)*deltT_DP + j*deltT_QP;
        % 位置
        ST_QP(idx,1) = T;
        ST_QP(idx,2) = coeff(i,1) + coeff(i,2)*t + coeff(i,3)*t^2 ...
            + coeff(i,4) * t^3 + coeff(i,5) * t^4 +coeff(i,6) * t^5;
        
        % 速度
        v_QP(idx,1) = T;
        v_QP(idx,2) = coeff(i,2) + 2*coeff(i,3)*t + 3*coeff(i,4) * t^2 + ...
            4*coeff(i,5) * t^3 + 5*coeff(i,6) * t^4;
        
        % 加速度
        a_QP(idx,1) = T;
        a_QP(idx,2) = 2*coeff(i,3) + 6*coeff(i,4) * t + ...
            12*coeff(i,5) * t^2 + 20*coeff(i,6) * t^3;
    end
end
